simulink library "tramontina_database_gnsslib"  (R2024a)
settings: Solver=VariableStepAuto  StartTime=0.0  StopTime=10.0  RelTol=1e-3
libraries: canmsglib x6, simulink x1
settings Model: Creator=matlab.cut  LastModifiedBy=matlab.cut

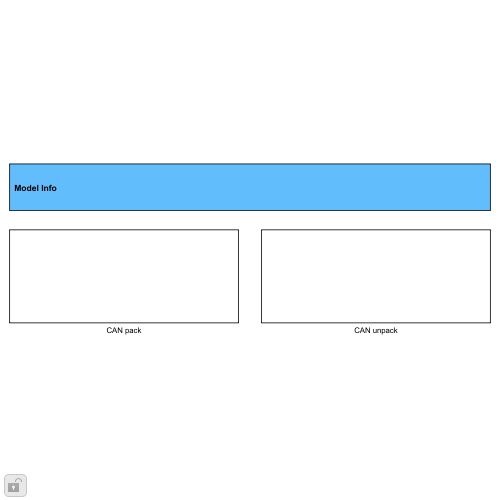
[thumbnail: Simulink's stored preview of the top-level diagram]
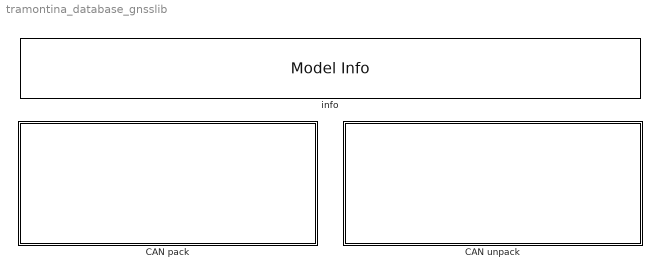
== system tramontina_database_gnsslib ==
  CAN pack : Subsystem
  CAN unpack : Subsystem
  info : simulink/Model-Wide Utilities/Model Info  Frame=on  DisplayStringWithTags=SPEEDGOAT CAN Database Library for: tramontina_database_gnss  HorizontalTextAlignment=Left  LeftAlignmentValue=0.01

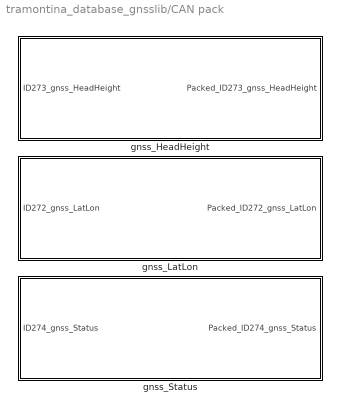
== system tramontina_database_gnsslib/CAN pack ==
  gnss_HeadHeight : Subsystem
  gnss_LatLon : Subsystem
  gnss_Status : Subsystem

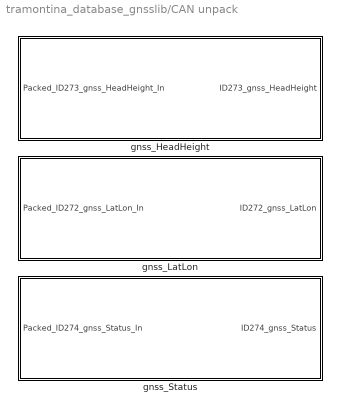
== system tramontina_database_gnsslib/CAN unpack ==
  gnss_HeadHeight : Subsystem
  gnss_LatLon : Subsystem
  gnss_Status : Subsystem

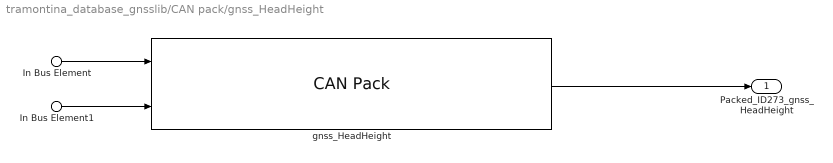
== system tramontina_database_gnsslib/CAN pack/gnss_HeadHeight ==
  In Bus Element : Inport  PortName=ID273_gnss_HeadHeight  Element=heading
  In Bus Element1 : Inport  PortName=ID273_gnss_HeadHeight  Element=height
  gnss_HeadHeight : canmsglib/CAN Pack  CANdbFile=C:\Users\matlab.cut\Desktop\matlab\AMR_tramontina\Data\DBCFiles\tramontina_database_gnss.dbc  MsgList=gnss_HeadHeight  MsgName=gnss_HeadHeight  MsgIDType=Standard (11-bit identifier)  MsgIdentifier=273  MsgLength=8  Remote=off  ApplyMinMax=off  BusOutput=on  SignalInfo={'heading','0','32','LE','signed','Standard','0','1','0','0','360';'height','32','32','LE','signed','Standard','0','1','0','-Inf','Inf'}
      settings: DataFormat=manually specified signals
  Packed_ID273_gnss_HeadHeight : Outport
  wires:
  gnss_HeadHeight/1 -> Packed_ID273_gnss_HeadHeight/1
  In Bus Element/1 -> gnss_HeadHeight/1
  In Bus Element1/1 -> gnss_HeadHeight/2

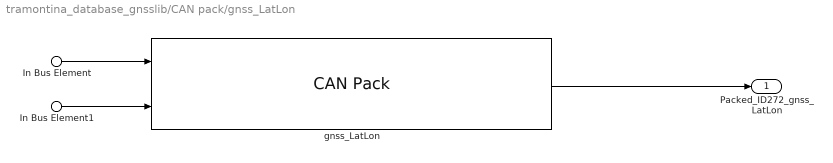
== system tramontina_database_gnsslib/CAN pack/gnss_LatLon ==
  In Bus Element : Inport  PortName=ID272_gnss_LatLon  Element=lat
  In Bus Element1 : Inport  PortName=ID272_gnss_LatLon  Element=lon
  gnss_LatLon : canmsglib/CAN Pack  CANdbFile=C:\Users\matlab.cut\Desktop\matlab\AMR_tramontina\Data\DBCFiles\tramontina_database_gnss.dbc  MsgList=gnss_LatLon  MsgName=gnss_LatLon  MsgIDType=Standard (11-bit identifier)  MsgIdentifier=272  MsgLength=8  Remote=off  ApplyMinMax=off  BusOutput=on  SignalInfo={'lat','0','32','LE','signed','Standard','0','1','0','-90','90';'lon','32','32','LE','signed','Standard','0','1','0','-180','180'}
      settings: DataFormat=manually specified signals
  Packed_ID272_gnss_LatLon : Outport
  wires:
  gnss_LatLon/1 -> Packed_ID272_gnss_LatLon/1
  In Bus Element/1 -> gnss_LatLon/1
  In Bus Element1/1 -> gnss_LatLon/2

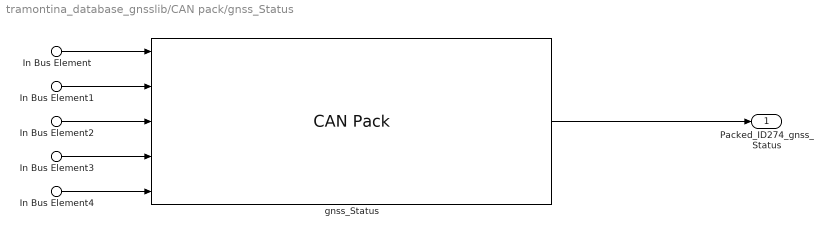
== system tramontina_database_gnsslib/CAN pack/gnss_Status ==
  In Bus Element : Inport  PortName=ID274_gnss_Status  Element=gnss_carr_soln_fixed
  In Bus Element1 : Inport  PortName=ID274_gnss_Status  Element=gnss_diff_soln
  In Bus Element2 : Inport  PortName=ID274_gnss_Status  Element=gnss_fix_ok
  In Bus Element3 : Inport  PortName=ID274_gnss_Status  Element=gnss_rel_pos_head_valid
  In Bus Element4 : Inport  PortName=ID274_gnss_Status  Element=numSV
  gnss_Status : canmsglib/CAN Pack  CANdbFile=C:\Users\matlab.cut\Desktop\matlab\AMR_tramontina\Data\DBCFiles\tramontina_database_gnss.dbc  MsgList=gnss_Status  MsgName=gnss_Status  MsgIDType=Standard (11-bit identifier)  MsgIdentifier=274  MsgLength=8  Remote=off  ApplyMinMax=off  BusOutput=on  SignalInfo={'gnss_carr_soln_fixed','10','1','LE','unsigned','Standard','0','1','0','-Inf','Inf';'gnss_diff_soln','9','1','LE','unsigned','Standard','0','1','0','-Inf','Inf';'gnss_fix_ok','8','1','LE','unsigned','Standard','0','1','0','-Inf','Inf';'gnss_rel_pos_head_valid','11','1','LE','unsigned','Standard','0','1','0','-Inf','Inf';'numSV','0','8','LE','unsigned','Standard','0','1','0','0','31'}
      settings: DataFormat=manually specified signals
  Packed_ID274_gnss_Status : Outport
  wires:
  gnss_Status/1 -> Packed_ID274_gnss_Status/1
  In Bus Element/1 -> gnss_Status/1
  In Bus Element1/1 -> gnss_Status/2
  In Bus Element2/1 -> gnss_Status/3
  In Bus Element3/1 -> gnss_Status/4
  In Bus Element4/1 -> gnss_Status/5

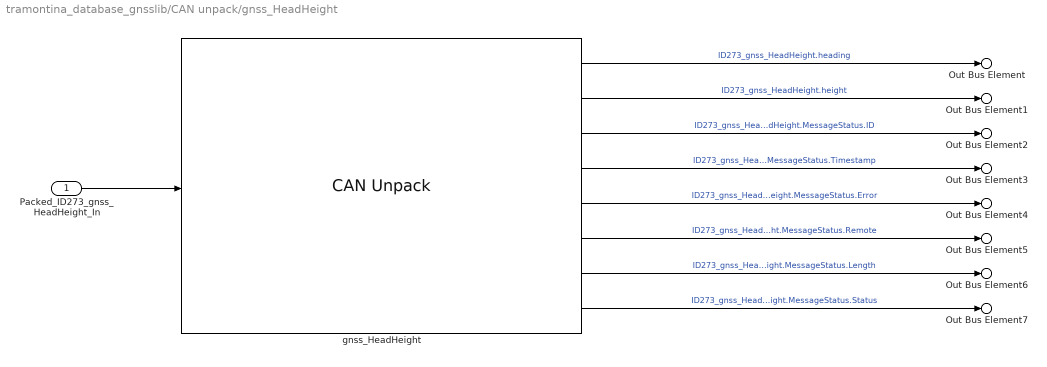
== system tramontina_database_gnsslib/CAN unpack/gnss_HeadHeight ==
  Packed_ID273_gnss_HeadHeight_In : Inport
  gnss_HeadHeight : canmsglib/CAN Unpack  CANdbFile=C:\Users\matlab.cut\Desktop\matlab\AMR_tramontina\Data\DBCFiles\tramontina_database_gnss.dbc  MsgList=gnss_HeadHeight  MsgName=gnss_HeadHeight  MsgIDType=Standard (11-bit identifier)  MsgIdentifier=273  MsgLength=8  SignalInfo={'heading','0','32','LE','signed','Standard','0','1','0','0','360';'height','32','32','LE','signed','Standard','0','1','0','-Inf','Inf'}  IDPort=on  TimestampPort=on  ErrorPort=on  RemotePort=on  LengthPort=on  StatusPort=on  ApplyMinMax=off
  Out Bus Element : Outport  PortName=ID273_gnss_HeadHeight  Element=heading
  Out Bus Element1 : Outport  PortName=ID273_gnss_HeadHeight  Element=height
  Out Bus Element2 : Outport  PortName=ID273_gnss_HeadHeight  Element=MessageStatus.ID
  Out Bus Element3 : Outport  PortName=ID273_gnss_HeadHeight  Element=MessageStatus.Timestamp
  Out Bus Element4 : Outport  PortName=ID273_gnss_HeadHeight  Element=MessageStatus.Error
  Out Bus Element5 : Outport  PortName=ID273_gnss_HeadHeight  Element=MessageStatus.Remote
  Out Bus Element6 : Outport  PortName=ID273_gnss_HeadHeight  Element=MessageStatus.Length
  Out Bus Element7 : Outport  PortName=ID273_gnss_HeadHeight  Element=MessageStatus.Status
  wires:
  Packed_ID273_gnss_HeadHeight_In/1 -> gnss_HeadHeight/1
  gnss_HeadHeight/1 -> Out Bus Element/1  "ID273_gnss_HeadHeight.heading"
  gnss_HeadHeight/2 -> Out Bus Element1/1  "ID273_gnss_HeadHeight.height"
  gnss_HeadHeight/3 -> Out Bus Element2/1  "ID273_gnss_HeadHeight.MessageStatus.ID"
  gnss_HeadHeight/4 -> Out Bus Element3/1  "ID273_gnss_HeadHeight.MessageStatus.Timestamp"
  gnss_HeadHeight/5 -> Out Bus Element4/1  "ID273_gnss_HeadHeight.MessageStatus.Error"
  gnss_HeadHeight/6 -> Out Bus Element5/1  "ID273_gnss_HeadHeight.MessageStatus.Remote"
  gnss_HeadHeight/7 -> Out Bus Element6/1  "ID273_gnss_HeadHeight.MessageStatus.Length"
  gnss_HeadHeight/8 -> Out Bus Element7/1  "ID273_gnss_HeadHeight.MessageStatus.Status"

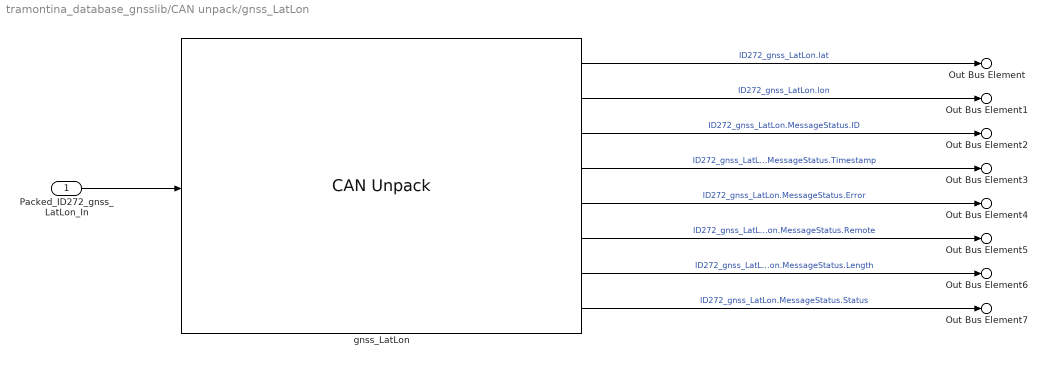
== system tramontina_database_gnsslib/CAN unpack/gnss_LatLon ==
  Packed_ID272_gnss_LatLon_In : Inport
  gnss_LatLon : canmsglib/CAN Unpack  CANdbFile=C:\Users\matlab.cut\Desktop\matlab\AMR_tramontina\Data\DBCFiles\tramontina_database_gnss.dbc  MsgList=gnss_LatLon  MsgName=gnss_LatLon  MsgIDType=Standard (11-bit identifier)  MsgIdentifier=272  MsgLength=8  SignalInfo={'lat','0','32','LE','signed','Standard','0','1','0','-90','90';'lon','32','32','LE','signed','Standard','0','1','0','-180','180'}  IDPort=on  TimestampPort=on  ErrorPort=on  RemotePort=on  LengthPort=on  StatusPort=on  ApplyMinMax=off
  Out Bus Element : Outport  PortName=ID272_gnss_LatLon  Element=lat
  Out Bus Element1 : Outport  PortName=ID272_gnss_LatLon  Element=lon
  Out Bus Element2 : Outport  PortName=ID272_gnss_LatLon  Element=MessageStatus.ID
  Out Bus Element3 : Outport  PortName=ID272_gnss_LatLon  Element=MessageStatus.Timestamp
  Out Bus Element4 : Outport  PortName=ID272_gnss_LatLon  Element=MessageStatus.Error
  Out Bus Element5 : Outport  PortName=ID272_gnss_LatLon  Element=MessageStatus.Remote
  Out Bus Element6 : Outport  PortName=ID272_gnss_LatLon  Element=MessageStatus.Length
  Out Bus Element7 : Outport  PortName=ID272_gnss_LatLon  Element=MessageStatus.Status
  wires:
  Packed_ID272_gnss_LatLon_In/1 -> gnss_LatLon/1
  gnss_LatLon/1 -> Out Bus Element/1  "ID272_gnss_LatLon.lat"
  gnss_LatLon/2 -> Out Bus Element1/1  "ID272_gnss_LatLon.lon"
  gnss_LatLon/3 -> Out Bus Element2/1  "ID272_gnss_LatLon.MessageStatus.ID"
  gnss_LatLon/4 -> Out Bus Element3/1  "ID272_gnss_LatLon.MessageStatus.Timestamp"
  gnss_LatLon/5 -> Out Bus Element4/1  "ID272_gnss_LatLon.MessageStatus.Error"
  gnss_LatLon/6 -> Out Bus Element5/1  "ID272_gnss_LatLon.MessageStatus.Remote"
  gnss_LatLon/7 -> Out Bus Element6/1  "ID272_gnss_LatLon.MessageStatus.Length"
  gnss_LatLon/8 -> Out Bus Element7/1  "ID272_gnss_LatLon.MessageStatus.Status"

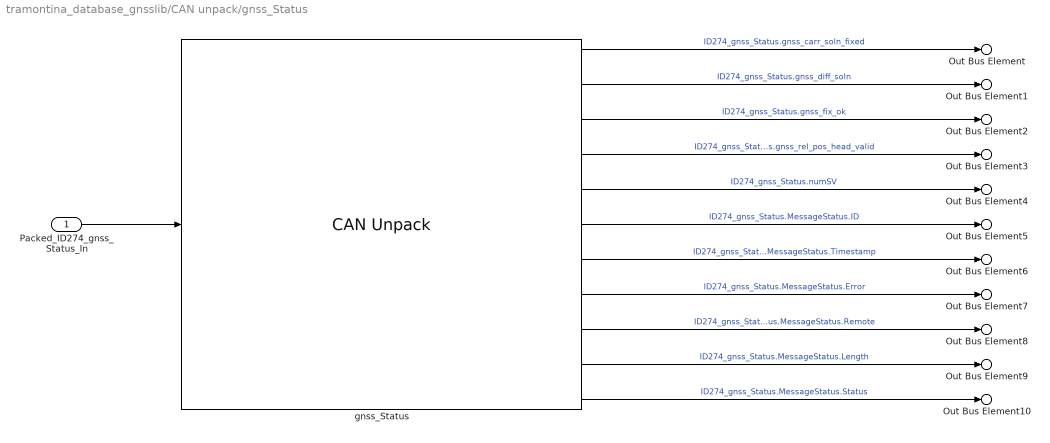
== system tramontina_database_gnsslib/CAN unpack/gnss_Status ==
  Packed_ID274_gnss_Status_In : Inport
  gnss_Status : canmsglib/CAN Unpack  CANdbFile=C:\Users\matlab.cut\Desktop\matlab\AMR_tramontina\Data\DBCFiles\tramontina_database_gnss.dbc  MsgList=gnss_Status  MsgName=gnss_Status  MsgIDType=Standard (11-bit identifier)  MsgIdentifier=274  MsgLength=8  SignalInfo={'gnss_carr_soln_fixed','10','1','LE','unsigned','Standard','0','1','0','-Inf','Inf';'gnss_diff_soln','9','1','LE','unsigned','Standard','0','1','0','-Inf','Inf';'gnss_fix_ok','8','1','LE','unsigned','Standard','0','1','0','-Inf','Inf';'gnss_rel_pos_head_valid','11','1','LE','unsigned','Standard','0','1','0','-Inf','Inf';'numSV','0','8','LE','unsigned','Standard','0','1','0','0','31'}  IDPort=on  TimestampPort=on  ErrorPort=on  RemotePort=on  LengthPort=on  StatusPort=on  ApplyMinMax=off
  Out Bus Element : Outport  PortName=ID274_gnss_Status  Element=gnss_carr_soln_fixed
  Out Bus Element1 : Outport  PortName=ID274_gnss_Status  Element=gnss_diff_soln
  Out Bus Element2 : Outport  PortName=ID274_gnss_Status  Element=gnss_fix_ok
  Out Bus Element3 : Outport  PortName=ID274_gnss_Status  Element=gnss_rel_pos_head_valid
  Out Bus Element4 : Outport  PortName=ID274_gnss_Status  Element=numSV
  Out Bus Element5 : Outport  PortName=ID274_gnss_Status  Element=MessageStatus.ID
  Out Bus Element6 : Outport  PortName=ID274_gnss_Status  Element=MessageStatus.Timestamp
  Out Bus Element7 : Outport  PortName=ID274_gnss_Status  Element=MessageStatus.Error
  Out Bus Element8 : Outport  PortName=ID274_gnss_Status  Element=MessageStatus.Remote
  Out Bus Element9 : Outport  PortName=ID274_gnss_Status  Element=MessageStatus.Length
  Out Bus Element10 : Outport  PortName=ID274_gnss_Status  Element=MessageStatus.Status
  wires:
  Packed_ID274_gnss_Status_In/1 -> gnss_Status/1
  gnss_Status/1 -> Out Bus Element/1  "ID274_gnss_Status.gnss_carr_soln_fixed"
  gnss_Status/2 -> Out Bus Element1/1  "ID274_gnss_Status.gnss_diff_soln"
  gnss_Status/3 -> Out Bus Element2/1  "ID274_gnss_Status.gnss_fix_ok"
  gnss_Status/4 -> Out Bus Element3/1  "ID274_gnss_Status.gnss_rel_pos_head_valid"
  gnss_Status/5 -> Out Bus Element4/1  "ID274_gnss_Status.numSV"
  gnss_Status/6 -> Out Bus Element5/1  "ID274_gnss_Status.MessageStatus.ID"
  gnss_Status/7 -> Out Bus Element6/1  "ID274_gnss_Status.MessageStatus.Timestamp"
  gnss_Status/8 -> Out Bus Element7/1  "ID274_gnss_Status.MessageStatus.Error"
  gnss_Status/9 -> Out Bus Element8/1  "ID274_gnss_Status.MessageStatus.Remote"
  gnss_Status/10 -> Out Bus Element9/1  "ID274_gnss_Status.MessageStatus.Length"
  gnss_Status/11 -> Out Bus Element10/1  "ID274_gnss_Status.MessageStatus.Status"
